simulink model "linear_sys"  (R2021b)
settings: Solver=ode4  StartTime=0  StopTime=T_end  FixedStep=dt  RelTol=1e-3
undefined symbols (not defined in the file or in its folder): IC, Kbbx, Kbby, PID_sim, ref, tau_mot_x, tau_mot_y, tau_sens_x, tau_sens_y, V2theta_x, V2theta_y
libraries: slpidlib x2
settings Model: Creator=Daniele Oranges  LastModifiedBy=ernesto
settings DataIOCC: SaveFormat=StructureWithTime
settings OptimizationCC: BlockReduction=off  BufferReuse=off
settings DebuggingCC: AlgebraicLoopMsg=none  UnconnectedInputMsg=none  UnconnectedOutputMsg=none  UnconnectedLineMsg=none
settings ExplorerConfigSet: SimMechanicsOpenEditorOnUpdate=off

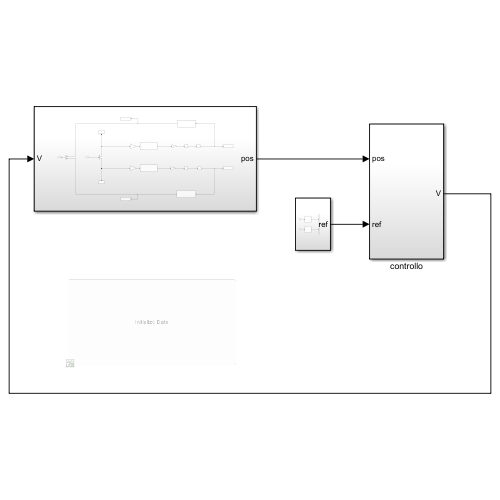
[thumbnail: Simulink's stored preview of the top-level diagram]
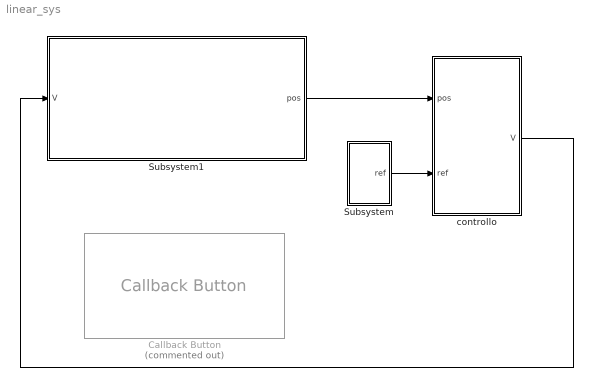
== system linear_sys ==
  Callback Button : CallbackButton  Commented=on  ButtonText=Initialize Data
      settings: ClickFcn=|
      | clear
      | data
  Subsystem : Subsystem
  Subsystem1 : Subsystem
  "controllo " : Subsystem
  wires:
  Subsystem/1(ref) -> "controllo "/2(ref)
  Subsystem1/1(pos) -> "controllo "/1("pos ")
  "controllo "/1(V) -> Subsystem1/1(V)

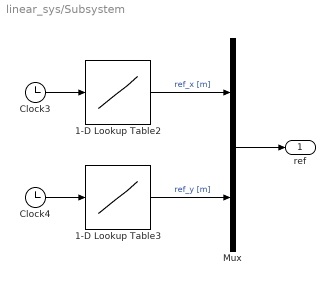
== system linear_sys/Subsystem ==
  1-D Lookup Table2 : Lookup_n-D  NumberOfTableDimensions=1  BreakpointsForDimension1=ref.x.t  Table=ref.x.v  InternalRulePriority=Speed  RndMeth=Simplest  InputSameDT=on
  1-D Lookup Table3 : Lookup_n-D  NumberOfTableDimensions=1  BreakpointsForDimension1=ref.y.t  Table=ref.y.v  InternalRulePriority=Speed  RndMeth=Simplest  InputSameDT=on
  Clock3 : Clock
  Clock4 : Clock
  Mux : Mux  Inputs=2
  ref : Outport
  wires:
  Mux/1 -> ref/1
  Clock4/1 -> 1-D Lookup Table3/1
  Clock3/1 -> 1-D Lookup Table2/1
  1-D Lookup Table3/1 -> Mux/2  "ref_y [m]"
  1-D Lookup Table2/1 -> Mux/1  "ref_x [m]"

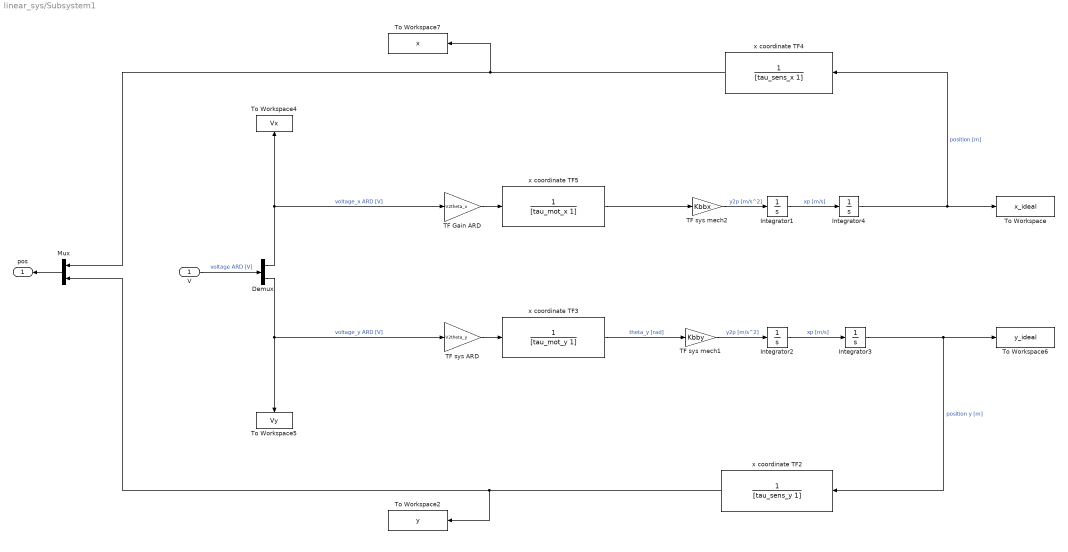
== system linear_sys/Subsystem1 ==
  V : Inport
  Demux : Demux  Outputs=2
  Integrator1 : Integrator
  Integrator2 : Integrator
  Integrator3 : Integrator  InitialCondition=IC(2)
  Integrator4 : Integrator  InitialCondition=IC(1)
  Mux : Mux  Inputs=2
  TF Gain ARD : Gain  Gain=V2theta_x
  TF sys ARD : Gain  Gain=V2theta_y
  TF sys mech1 : Gain  Gain=Kbby
  TF sys mech2 : Gain  Gain=Kbbx
  To Workspace : ToWorkspace  VariableName=x_ideal  SaveFormat=Timeseries  SampleTime=-1
  To Workspace2 : ToWorkspace  VariableName=y  SaveFormat=Timeseries  SampleTime=-1
  To Workspace4 : ToWorkspace  VariableName=Vx  SaveFormat=Timeseries  SampleTime=-1
  To Workspace5 : ToWorkspace  VariableName=Vy  SaveFormat=Timeseries  SampleTime=-1
  To Workspace6 : ToWorkspace  VariableName=y_ideal  SaveFormat=Timeseries  SampleTime=-1
  To Workspace7 : ToWorkspace  VariableName=x  SaveFormat=Timeseries  SampleTime=-1
  x coordinate TF2 : TransferFcn  Denominator=[tau_sens_y 1]
  x coordinate TF3 : TransferFcn  Denominator=[tau_mot_y 1]
  x coordinate TF4 : TransferFcn  Denominator=[tau_sens_x 1]
  x coordinate TF5 : TransferFcn  Denominator=[tau_mot_x 1]
  pos : Outport
  wires:
  Demux/1 -> TF Gain ARD/1, To Workspace4/1  "voltage_x ARD [V]"
  Integrator4/1 -> To Workspace/1, x coordinate TF4/1  "position [m]"
  Demux/2 -> TF sys ARD/1, To Workspace5/1  "voltage_y ARD [V]"
  Integrator3/1 -> To Workspace6/1, x coordinate TF2/1  "position y [m]"
  V/1 -> Demux/1  "voltage ARD [V]"
  Mux/1 -> pos/1
  TF Gain ARD/1 -> x coordinate TF5/1
  x coordinate TF3/1 -> TF sys mech1/1  "theta_y [rad]"
  TF sys ARD/1 -> x coordinate TF3/1
  Integrator2/1 -> Integrator3/1  "xp [m/s]"
  TF sys mech1/1 -> Integrator2/1  "y2p [m/s^2]"
  Integrator1/1 -> Integrator4/1  "xp [m/s]"
  TF sys mech2/1 -> Integrator1/1  "y2p [m/s^2]"
  x coordinate TF2/1 -> To Workspace2/1, Mux/2
  x coordinate TF4/1 -> To Workspace7/1, Mux/1
  x coordinate TF5/1 -> TF sys mech2/1

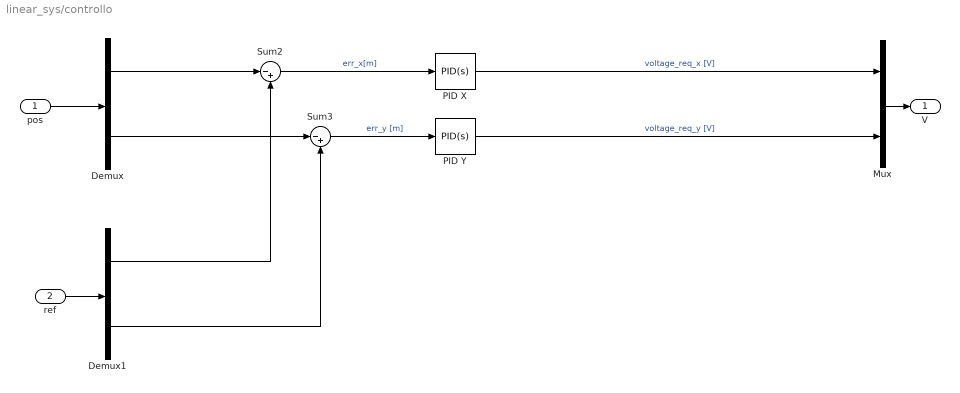
== system linear_sys/controllo  ==
  "pos " : Inport
  ref : Inport  Port=2
  Demux : Demux  Outputs=2
  Demux1 : Demux  Outputs=2
  Mux : Mux  Inputs=2
  PID X : slpidlib/PID Controller  Controller=PID  Form=Parallel  TimeDomain=Continuous-time  UseExternalTs=off  SampleTime=-1  IntegratorMethod=Forward Euler  FilterMethod=Forward Euler  ControllerParametersSource=internal  P=PID_sim.x.Kp  I=PID_sim.x.Ki  D=PID_sim.x.Kd  UseFilter=on  N=PID_sim.x.filter  TunerSelectOption=Transfer Function Based (PID Tuner App)  InitialConditionSource=internal  InitialConditionForIntegrator=0  InitialConditionForFilter=0  DifferentiatorICPrevScaledInput=0  ExternalReset=none  TrackingMode=off  Kt=1  LimitOutput=off  SatLimitsSource=internal  UpperSaturationLimit=inf  LowerSaturationLimit=-inf  LinearizeAsGain=on  AntiWindupMode=none  Kb=1  POutMin=[]  POutMax=[]  IOutMin=[]  IOutMax=[]  DOutMin=[]  DOutMax=[]  NOutMin=[]  NOutMax=[]  SumOutMin=[]  SumOutMax=[]  SaturationOutMin=[]  SaturationOutMax=[]  PParamMin=[]  PParamMax=[]  IParamMin=[]  IParamMax=[]  DParamMin=[]  DParamMax=[]  NParamMin=[]  NParamMax=[]  KbParamMin=[]  KbParamMax=[]  KtParamMin=[]  KtParamMax=[]  KbOutMin=[]  KbOutMax=[]  KtOutMin=[]  KtOutMax=[]  IntegratorOutMin=[]  IntegratorOutMax=[]  FilterOutMin=[]  FilterOutMax=[]  SumI1OutMin=[]  SumI1OutMax=[]  SumI2OutMin=[]  SumI2OutMax=[]  SumI3OutMin=[]  SumI3OutMax=[]  SumI4OutMin=[]  SumI4OutMax=[]  SumDOutMin=[]  SumDOutMax=[]  DifferentiatorOutMin=[]  DifferentiatorOutMax=[]  FilterDiffOutCoefMin=[]  FilterDiffOutCoefMax=[]  ReciprocalOutMin=[]  ReciprocalOutMax=[]  SumDenOutMin=[]  SumDenOutMax=[]  SumNumOutMin=[]  SumNumOutMax=[]  DivideOutMin=[]  DivideOutMax=[]  UdiffTsProdOutMin=[]  UdiffTsProdOutMax=[]  NTsProdOutMin=[]  NTsProdOutMax=[]  UintegralTsProdOutMin=[]  UintegralTsProdOutMax=[]  UngainTsProdOutMin=[]  UngainTsProdOutMax=[]  IntegratorContinuousStateAttributes=''  IntegratorStateMustResolveToSignalObject=off  IntegratorRTWStateStorageClass=Auto  FilterContinuousStateAttributes=''  FilterStateMustResolveToSignalObject=off  FilterRTWStateStorageClass=Auto  ParallelPVariant=InternalParameters  IdealPVariant=Disabled  IVariant=InternalParameters  DVariant=InternalParameters  IntegratorVariant=Continuous  SatVariant=Disabled  AWVariant=Passthrough  PCopyVariant=Disabled  TRVariant=Disabled  FdbkBlocksVariant=Forward  IdealPFdbkVariant=Disabled  SatFdbkVariant=Disabled  DerivativeFilterVariant=ContFilter  NVariant=InternalParameters  NCopyVariant=Disabled  FilterICVariant=InternalICsFilter  IntegratorICVariant=InternalICs  ExternalResetVariant=Disabled  TRSumVariant=Passthrough  SumFdbkVariant=Disabled  SumVariant=Sum_PID  TsampFilterVariant=InternalTs  TsampNgainVariant=Passthrough  TsampIntegralVariant=Passthrough  ExternalSaturationOutDataTypeStr=Inherit: Same as second input
  PID Y : slpidlib/PID Controller  Controller=PID  Form=Parallel  TimeDomain=Continuous-time  UseExternalTs=off  SampleTime=-1  IntegratorMethod=Forward Euler  FilterMethod=Forward Euler  ControllerParametersSource=internal  P=PID_sim.y.Kp  I=PID_sim.y.Ki  D=PID_sim.y.Kd  UseFilter=on  N=PID_sim.y.filter  TunerSelectOption=Transfer Function Based (PID Tuner App)  InitialConditionSource=internal  InitialConditionForIntegrator=0  InitialConditionForFilter=0  DifferentiatorICPrevScaledInput=0  ExternalReset=none  TrackingMode=off  Kt=1  LimitOutput=off  SatLimitsSource=internal  UpperSaturationLimit=inf  LowerSaturationLimit=-inf  LinearizeAsGain=on  AntiWindupMode=none  Kb=1  POutMin=[]  POutMax=[]  IOutMin=[]  IOutMax=[]  DOutMin=[]  DOutMax=[]  NOutMin=[]  NOutMax=[]  SumOutMin=[]  SumOutMax=[]  SaturationOutMin=[]  SaturationOutMax=[]  PParamMin=[]  PParamMax=[]  IParamMin=[]  IParamMax=[]  DParamMin=[]  DParamMax=[]  NParamMin=[]  NParamMax=[]  KbParamMin=[]  KbParamMax=[]  KtParamMin=[]  KtParamMax=[]  KbOutMin=[]  KbOutMax=[]  KtOutMin=[]  KtOutMax=[]  IntegratorOutMin=[]  IntegratorOutMax=[]  FilterOutMin=[]  FilterOutMax=[]  SumI1OutMin=[]  SumI1OutMax=[]  SumI2OutMin=[]  SumI2OutMax=[]  SumI3OutMin=[]  SumI3OutMax=[]  SumI4OutMin=[]  SumI4OutMax=[]  SumDOutMin=[]  SumDOutMax=[]  DifferentiatorOutMin=[]  DifferentiatorOutMax=[]  FilterDiffOutCoefMin=[]  FilterDiffOutCoefMax=[]  ReciprocalOutMin=[]  ReciprocalOutMax=[]  SumDenOutMin=[]  SumDenOutMax=[]  SumNumOutMin=[]  SumNumOutMax=[]  DivideOutMin=[]  DivideOutMax=[]  UdiffTsProdOutMin=[]  UdiffTsProdOutMax=[]  NTsProdOutMin=[]  NTsProdOutMax=[]  UintegralTsProdOutMin=[]  UintegralTsProdOutMax=[]  UngainTsProdOutMin=[]  UngainTsProdOutMax=[]  IntegratorContinuousStateAttributes=''  IntegratorStateMustResolveToSignalObject=off  IntegratorRTWStateStorageClass=Auto  FilterContinuousStateAttributes=''  FilterStateMustResolveToSignalObject=off  FilterRTWStateStorageClass=Auto  ParallelPVariant=InternalParameters  IdealPVariant=Disabled  IVariant=InternalParameters  DVariant=InternalParameters  IntegratorVariant=Continuous  SatVariant=Disabled  AWVariant=Passthrough  PCopyVariant=Disabled  TRVariant=Disabled  FdbkBlocksVariant=Forward  IdealPFdbkVariant=Disabled  SatFdbkVariant=Disabled  DerivativeFilterVariant=ContFilter  NVariant=InternalParameters  NCopyVariant=Disabled  FilterICVariant=InternalICsFilter  IntegratorICVariant=InternalICs  ExternalResetVariant=Disabled  TRSumVariant=Passthrough  SumFdbkVariant=Disabled  SumVariant=Sum_PID  TsampFilterVariant=InternalTs  TsampNgainVariant=Passthrough  TsampIntegralVariant=Passthrough  ExternalSaturationOutDataTypeStr=Inherit: Same as second input
  Sum2 : Sum  Inputs=|-+
  Sum3 : Sum  Inputs=|-+
  V : Outport
  wires:
  "pos "/1 -> Demux/1
  Mux/1 -> V/1
  Demux/1 -> Sum2/1
  Demux/2 -> Sum3/1
  PID X/1 -> Mux/1  "voltage_req_x [V]"
  Sum2/1 -> PID X/1  "err_x[m]"
  Sum3/1 -> PID Y/1  "err_y [m]"
  PID Y/1 -> Mux/2  "voltage_req_y [V]"
  Demux1/1 -> Sum2/2
  Demux1/2 -> Sum3/2
  ref/1 -> Demux1/1
